simulink model "heater_on_off"  (R2024b)
settings: Solver=VariableStepAuto  StartTime=0.0  StopTime=10.0  RelTol=1e-3
values from neighbouring files (symbols this model uses):
  C = 10    [heater_params.m]
  k = 1    [heater_params.m]
  T0 = 0    [heater_params.m]
settings Model: Creator=martinhaugen  LastModifiedBy=martinhaugen

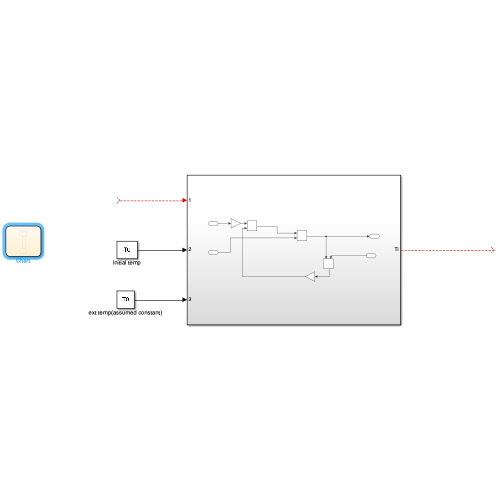
[thumbnail: Simulink's stored preview of the top-level diagram]
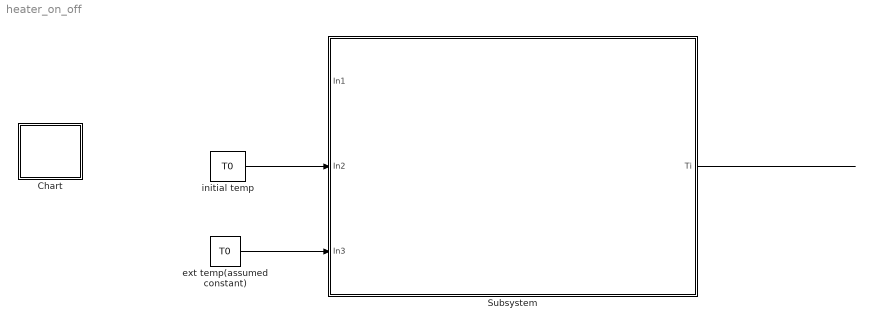
== system heater_on_off ==
  Chart : Stateflow chart  TreatAsAtomicUnit=on
  Subsystem : Subsystem
  ext temp(assumed constant) : Constant  Value=T0
  initial temp : Constant  Value=T0
  wires:
  ? -> Subsystem/1(In1)
  initial temp/1 -> Subsystem/2(In2)
  ext temp(assumed constant)/1 -> Subsystem/3(In3)
  Subsystem/1(Ti) -> ?

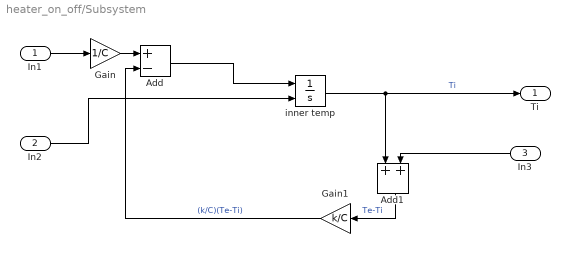
== system heater_on_off/Subsystem ==
  In1 : Inport
  In2 : Inport  Port=2
  In3 : Inport  Port=3
  Add : Sum  Inputs=+-
  Add1 : Sum
  Gain : Gain  Gain=1/C
  Gain1 : Gain  Gain=k/C
  inner temp : Integrator  InitialConditionSource=external
  Ti : Outport
  wires:
  In3/1 -> Add1/2
  In2/1 -> inner temp/2
  Gain/1 -> Add/1
  In1/1 -> Gain/1
  inner temp/1 -> Ti/1, Add1/1  "Ti"
  Add/1 -> inner temp/1
  Gain1/1 -> Add/2  "(k/C)(Te-Ti)"
  Add1/1 -> Gain1/1  "Te-Ti"

== stateflow chart heater_on_off/Chart ==
  state HEATING
    entry:
    u=1;
  state COOLING
    entry:
    u=0;
  (default) -> HEATING
  COOLING -> HEATING
  HEATING -> COOLING
